simulink model "EV_Modeling"  (R2024b)
(part 3 of 9)

  SOC-Vol/1 -> Voltage_cell/1, " Normalization"/2(Voltage), Vol-R/1, Divide11/1, Vol_pack/1  "Vsoc"
  Gain5/1 -> Compare To Constant/1, Battery_SOC[%]/1, SOC switch/1  "LSTM_FV1"
  Compare To Constant/1 -> Stop Simulation/1
  Step/1 -> SOC switch/2
